simulink model "Lead_Compensator_code (2)"  (R2021a)
settings: Solver=VariableStepAuto  StartTime=0.0  StopTime=2  RelTol=1e-3
libraries: simulink x2
settings Model: Creator=Electrical Dept  LastModifiedBy=mofid
settings SolverCC: AlgebraicLoopSolver=TrustRegion
settings SFSimCC: CustomCodeUndefinedFunction=UseInterfaceOnly
settings RTWCC: DLArmComputeVersion=20.02.1

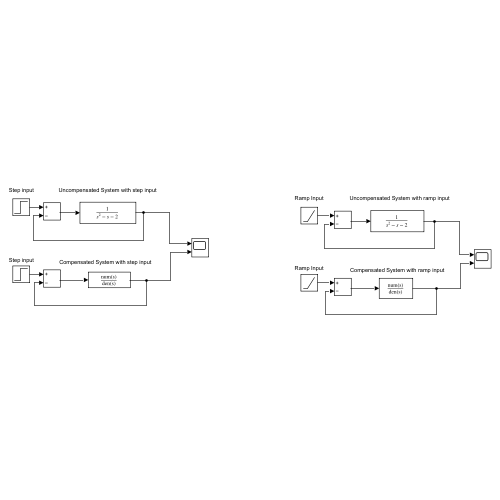
[thumbnail: Simulink's stored preview of the top-level diagram]
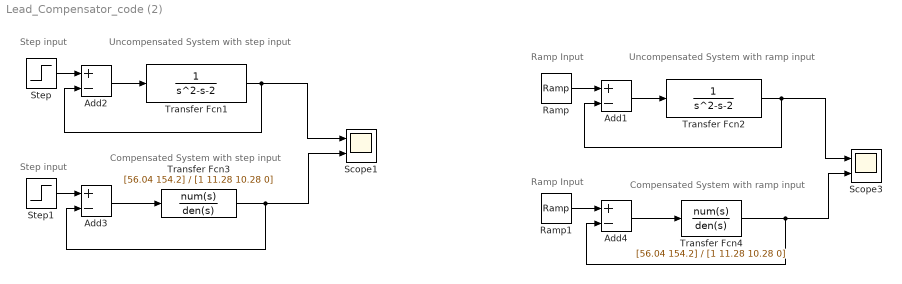
== system Lead_Compensator_code (2) ==
  note: Ramp Input
  note: Step input
  note: Compensated System with step input
  note: Uncompensated System with step input
  note: Compensated System with ramp input
  note: Uncompensated System with ramp input
  note: Step input
  note: Ramp Input
  Add{1..4} (4 alike) : Sum  Inputs=+-
  Ramp : simulink/Sources/Ramp  slope=1  start=0  InitialOutput=0
  Ramp1 : simulink/Sources/Ramp  slope=1  start=0  InitialOutput=0
  Scope1 : Scope  NumInputPorts=2
  Scope3 : Scope  NumInputPorts=2
  Step : Step  Time=0  SampleTime=0
  Step1 : Step  Time=0  SampleTime=0
  Transfer Fcn1 : TransferFcn  Denominator=[1 -1 -2]
  Transfer Fcn2 : TransferFcn  Denominator=[1 -1 -2]
  Transfer Fcn3 : TransferFcn  Numerator=[56.04 154.2]  Denominator=[1 11.28 10.28 0]
  Transfer Fcn4 : TransferFcn  Numerator=[56.04 154.2]  Denominator=[1 11.28 10.28 0]
  wires:
  Add2/1 -> Transfer Fcn1/1
  Transfer Fcn1/1 -> Add2/2, Scope1/1
  Transfer Fcn3/1 -> Scope1/2, Add3/2
  Add3/1 -> Transfer Fcn3/1
  Step/1 -> Add2/1
  Step1/1 -> Add3/1
  Ramp1/1 -> Add4/1
  Ramp/1 -> Add1/1
  Add4/1 -> Transfer Fcn4/1
  Transfer Fcn4/1 -> Add4/2, Scope3/2
  Transfer Fcn2/1 -> Add1/2, Scope3/1
  Add1/1 -> Transfer Fcn2/1
